simulink model "s9_template"  (R2023b)
settings: Solver=ode4  StartTime=0.0  StopTime=inf  FixedStep=P_sim_dt  RelTol=1e-3
InitFcn:
  | %madctrl_data;
  | s6_data;
values from neighbouring files (symbols this model uses):
  a1total = 2.70    (= 2.7)    [s6_data.m]
  a2total = 1.8    [s6_data.m]
  CarInputsCmdForward = uint8(1)    [p_mad_car.m]
  CarInputsCmdHalt = uint8(0)    [p_mad_car.m]
  CarInputsCmdReverse = uint8(2)    [p_mad_car.m]
  CarInputsCmdSlow = uint8(3)    [p_mad_car.m]
  P_k_p = 1    [s6_data.m]
  P_kr = 0.3440    (= 0.344)    [s6_data.m]
  P_ManeuverTypePark = 1    [s6_data.m]
  P_ManeuverTypePathFollow = 0    [s6_data.m]
  P_p_Bf = 0.7    [p_mad_car.m]
  P_p_Br = 0.7    [p_mad_car.m]
  P_p_Cf = 2    [p_mad_car.m]
  P_p_Cr = 2    [p_mad_car.m]
  P_p_delta_max = 21.58/180*pi    (= 0.37664205258)    [p_mad_car.m]
  P_p_Df = 2    [p_mad_car.m]
  P_p_Dr = 2.5    [p_mad_car.m]
  P_p_Ef = -0.1    [p_mad_car.m]
  P_p_Er = -0.05    [p_mad_car.m]
  P_p_J = 192e-6    (= 0.000192)    [p_mad_car.m]
  P_p_k = 2.51    [p_mad_car.m]
  P_p_l = abs(P_p_frontaxle_1 + P_p_rearaxle_1)    [p_mad_car.m]
  P_p_lf = P_p_frontaxle_1    (= 0.05)    [p_mad_car.m]
  P_p_lr = P_p_rearaxle_1    (= 0.049)    [p_mad_car.m]
  P_p_m = 132e-3    (= 0.132)    [p_mad_car.m]
  P_p_own = [P_p_s10; P_p_s20; 0; 0; 0; 0; 0 ]    [p_mad_car.m]
  P_p_T = 316e-3    (= 0.316)    [p_mad_car.m]
  P_p_Tt = P_p_uTt + P_p_output_Tt    (= 0.1)    [p_mad_car.m]
  P_p_Tw = 300e-3    (= 0.3)    [s6_data.m]
  P_prevent_buffer = 0.1    [s6_data.m]
  P_safety_buffer = 0.05    [s6_data.m]
  P_Ta = 20e-3    (= 0.02)    [s6_data.m]
  P_Ti = 0.2468    [s6_data.m]
  P_w_breakslen = uint32(length(path.points))    [s6_data.m]
  P_w_coefs = zeros(SPLINE.Elements(3).Dimensions)    [s6_data.m]
  P_w_points = zeros(SPLINE.Elements(2).Dimensions)    [s6_data.m]
  P_w_segments = uint32(zeros(SPLINE.Elements(4).Dimensions))    [s6_data.m]
  P_xManeuverEnd = 1    [s6_data.m]
  points = [p.x+x; s1; s2]    [mbc_clothoid_get_points.m]
undefined symbols (not defined in the file or in its folder): breakslen, coefs, DiscIntNeverNeededParam, periodic, segments
libraries: mad_lib_template x1, simulink x1
(part 1 of 2)
settings Model: Creator=hmekiedj  LastModifiedBy=Dominik
settings DataIOCC: ReturnWorkspaceOutputs=off
settings OptimizationCC: BlockReduction=off  DefaultParameterBehavior=Inlined  BufferReuse=off
settings DebuggingCC: UnconnectedInputMsg=warning  UnconnectedOutputMsg=warning  UnconnectedLineMsg=warning  ArithmeticOperatorsInVariantConditions=warning
settings ModelReferenceCC: EnableRefExpFcnMdlSchedulingChecks=on
settings SFSimCC: SimUseLocalCustomCode=off  CustomCodeUndefinedFunction=UseInterfaceOnly
settings RTWCC: RTWUseLocalCustomCode=off  DLArmComputeVersion=19.05
settings CodeAppCC: StateflowObjectComments=on

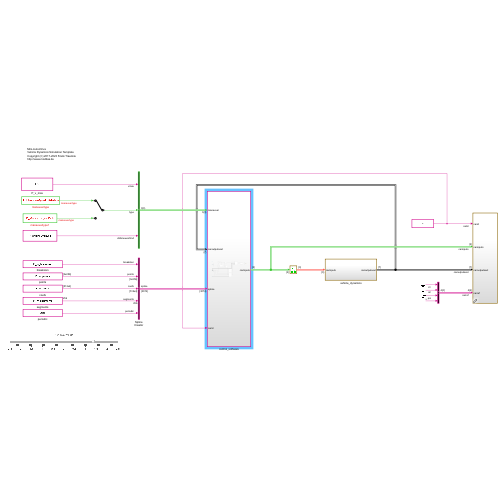
[thumbnail: Simulink's stored preview of the top-level diagram]
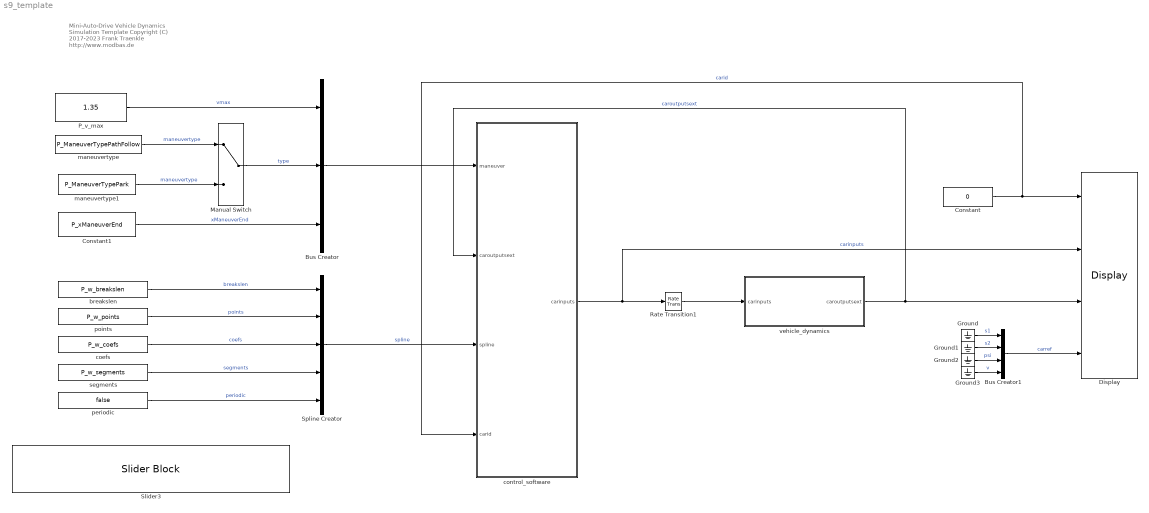
== system s9_template ==
  note: Mini-Auto-Drive
      | Vehicle Dynamics Simulation Template
      | Copyright (C) 2017-2023 Frank Traenkle
      | http://www.modbas.de
  Bus Creator : BusCreator  Inputs=3
  Bus Creator1 : BusCreator  Inputs=4
  Constant : Constant  Value=0
  Constant1 : Constant  Value=P_xManeuverEnd
  Display : mad_lib_template/Display  SystemSampleTime=-1  VariantActivationTime=update diagram  AllowFlexibleInterface=on  Latency=0  AutoFrameSizeCalculation=off
  Ground{,1..3} (4 alike) : Ground
  Manual Switch : ManualSwitch
  P_v_max : Constant  Value=1.35
  Rate Transition1 : RateTransition
  Slider3 : SliderBlock  ScaleMin=-2.50  ScaleMax=2.50  TickInterval=0.5
  Spline Creator : BusCreator  Inputs=breakslen,points,coefs,segments,periodic  OutDataTypeStr=Bus: SPLINE
  breakslen : Constant  Value=P_w_breakslen
  coefs : Constant  Value=P_w_coefs
  control_software : Subsystem  TreatAsAtomicUnit=on  SystemSampleTime=P_Ta
  maneuvertype : Constant  Value=P_ManeuverTypePathFollow  SampleTime=-1
  maneuvertype1 : Constant  Value=P_ManeuverTypePark  SampleTime=-1
  periodic : Constant  Value=false
  points : Constant  Value=P_w_points
  segments : Constant  Value=P_w_segments
  vehicle_dynamics : Subsystem
  wires:
  Bus Creator1/1 -> Display/4  "carref"
  Ground/1 -> Bus Creator1/1  "s1"
  Ground1/1 -> Bus Creator1/2  "s2"
  Ground2/1 -> Bus Creator1/3  "psi"
  Ground3/1 -> Bus Creator1/4  "v"
  vehicle_dynamics/1(caroutputsext) -> control_software/2(caroutputsext), Display/3  "caroutputsext"
  Rate Transition1/1 -> vehicle_dynamics/1(carinputs)
  control_software/1(carinputs) -> Display/2, Rate Transition1/1  "carinputs"
  Bus Creator/1 -> control_software/1(maneuver)
  P_v_max/1 -> Bus Creator/1  "vmax"
  Manual Switch/1 -> Bus Creator/2  "type"
  maneuvertype/1 -> Manual Switch/1  "maneuvertype"
  maneuvertype1/1 -> Manual Switch/2  "maneuvertype"
  Constant1/1 -> Bus Creator/3  "xManeuverEnd"
  periodic/1 -> Spline Creator/5  "periodic"
  coefs/1 -> Spline Creator/3  "coefs"
  points/1 -> Spline Creator/2  "points"
  breakslen/1 -> Spline Creator/1  "breakslen"
  segments/1 -> Spline Creator/4  "segments"
  Spline Creator/1 -> control_software/3(spline)  "spline"
  Constant/1 -> Display/1, control_software/4(carid)  "carid"

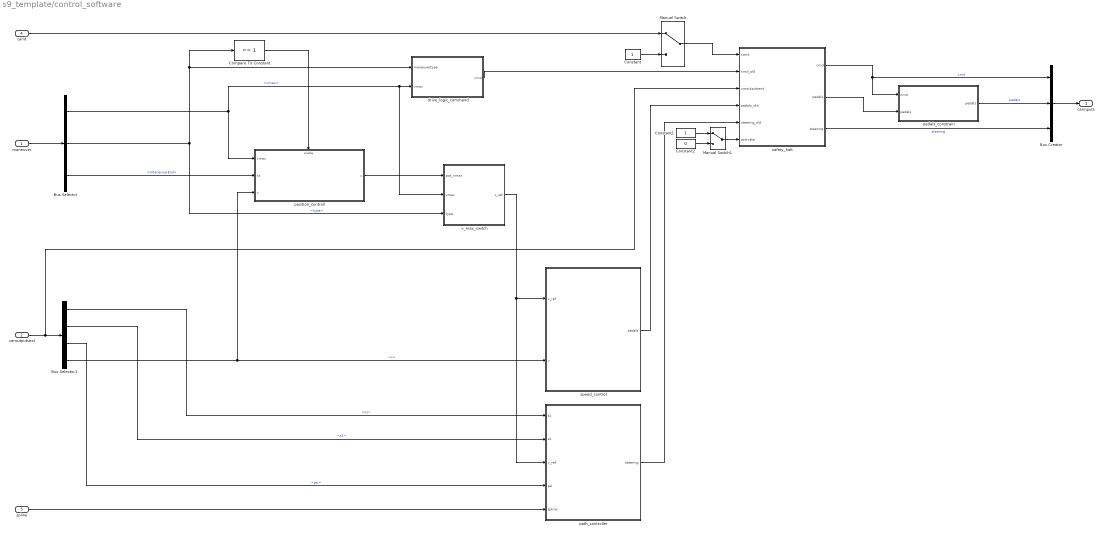
== system s9_template/control_software ==
  maneuver : Inport
  caroutputsext : Inport  Port=2
  spline : Inport  Port=3
  carid : Inport  Port=4
  Bus Creator : BusCreator  Inputs=3
  Bus Selector : BusSelector  OutputSignals=vmax,type,xManeuverEnd
  Bus Selector1 : BusSelector  OutputSignals=s1,s2,psi,v
  Compare To Constant : simulink/Logic and Bit Operations/Compare To Constant  relop===  const=1  OutDataTypeStr=boolean
  Constant : Constant
  Constant1 : Constant
  Constant2 : Constant  Value=0
  Manual Switch : ManualSwitch
  Manual Switch1 : ManualSwitch
  drive_logic_command : MATLAB Function  TreatAsAtomicUnit=on
  path_controller : Subsystem
  pedals_constrain : MATLAB Function  TreatAsAtomicUnit=on
  position_controll : Subsystem  TreatAsAtomicUnit=on
  safety_halt : MATLAB Function  TreatAsAtomicUnit=on
  speed_control : Subsystem
  v_max_switch : MATLAB Function  TreatAsAtomicUnit=on
  carinputs : Outport
  wires:
  caroutputsext/1 -> safety_halt/3(caroutputsext), Bus Selector1/1
  position_controll/1(u) -> v_max_switch/1(pos_vmax)
  maneuver/1 -> Bus Selector/1
  Bus Selector/1 -> position_controll/1(vmax), v_max_switch/2(vmax), drive_logic_command/2(vmax)  "<vmax>"
  Bus Selector/2 -> v_max_switch/3(type), Compare To Constant/1, drive_logic_command/1(maneuvertype)  "<type>"
  Compare To Constant/1 -> position_controll/Enable
  Bus Creator/1 -> carinputs/1
  Bus Selector/3 -> position_controll/2(xs)  "<xManeuverEnd>"
  drive_logic_command/1(cmd) -> safety_halt/2(cmd_old)
  path_controller/1(steering) -> safety_halt/5(steering_old)
  spline/1 -> path_controller/5(spline)
  safety_halt/1(cmd) -> pedals_constrain/1(cmd), Bus Creator/1  "cmd"
  carid/1 -> Manual Switch/1
  Bus Selector1/1 -> path_controller/1(s1)  "<s1>"
  Bus Selector1/2 -> path_controller/2(s2)  "<s2>"
  Bus Selector1/3 -> path_controller/4(psi)  "<psi>"
  Bus Selector1/4 -> position_controll/3(v), speed_control/2(v)  "<v>"
  Constant/1 -> Manual Switch/2
  Manual Switch/1 -> safety_halt/1(carid)
  v_max_switch/1(v_ref) -> path_controller/3(v_ref), speed_control/1(v_ref)
  speed_control/1(pedals) -> safety_halt/4(pedals_old)
  pedals_constrain/1(pedals) -> Bus Creator/2  "pedals"
  safety_halt/3(steering) -> Bus Creator/3  "steering"
  safety_halt/2(pedals) -> pedals_constrain/2("pedals ")
  Constant1/1 -> Manual Switch1/1
  Constant2/1 -> Manual Switch1/2
  Manual Switch1/1 -> safety_halt/6(activate)

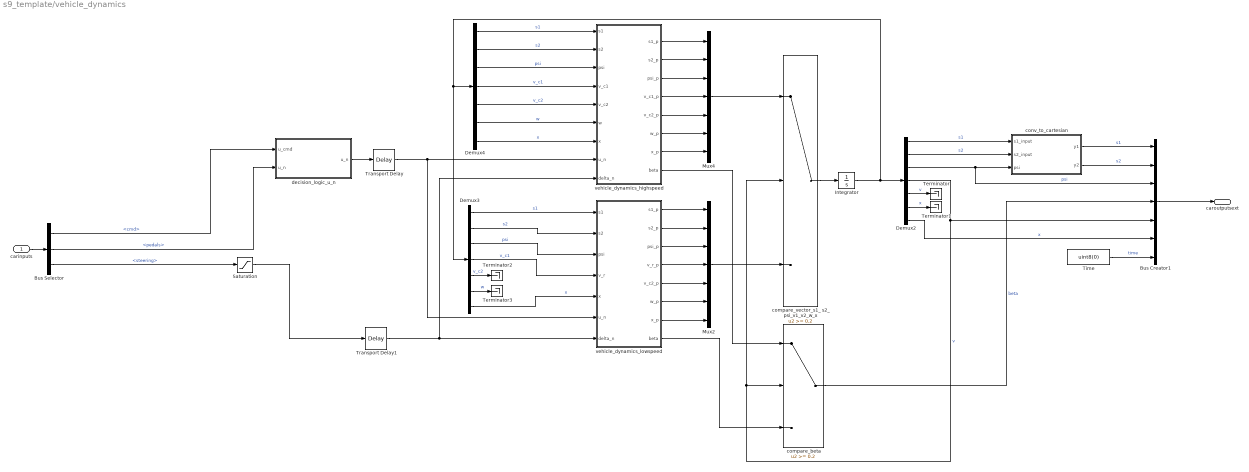
== system s9_template/vehicle_dynamics ==
  carinputs : Inport
  Bus Creator1 : BusCreator  Inputs=7  OutDataTypeStr=Bus: CAROUTPUTSEXT
  Bus Selector : BusSelector  OutputSignals=cmd,pedals,steering
  Demux2 : Demux  Outputs=7
  Demux3 : Demux  Outputs=7
  Demux4 : Demux  Outputs=7
  Integrator : Integrator  InitialCondition=P_p_own
  Mux2 : Mux  Inputs=7
  Mux4 : Mux  Inputs=7
  Saturation : Saturate  UpperLimit=1  LowerLimit=-1
  Terminator{,1..3} (4 alike) : Terminator
  Time : Constant  Value=uint8(0)
  Transport Delay : TransportDelay  DelayTime=P_p_Tt
  Transport Delay1 : TransportDelay  DelayTime=P_p_Tt
  compare_beta : Switch  Threshold=0.2  SaturateOnIntegerOverflow=off  InputSameDT=off
  compare_vector_s1_ s2_psi_v1_v2_w_x : Switch  Threshold=0.2  SaturateOnIntegerOverflow=off  InputSameDT=off
  conv_to_cartesian : MATLAB Function  TreatAsAtomicUnit=on
  decision_logic_u_n : MATLAB Function  TreatAsAtomicUnit=on
  vehicle_dynamics_highspeed : Subsystem
  vehicle_dynamics_lowspeed : Subsystem
  caroutputsext : Outport  VectorParamsAs1DForOutWhenUnconnected=off
  wires:
  carinputs/1 -> Bus Selector/1
  Bus Selector/2 -> decision_logic_u_n/2("u_n ")  "<pedals>"
  Bus Selector/3 -> Saturation/1  "<steering>"
  Demux2/3 -> conv_to_cartesian/3(psi), Bus Creator1/3  "psi"
  Bus Creator1/1 -> caroutputsext/1
  Demux2/7 -> Bus Creator1/6  "x"
  Demux2/2 -> conv_to_cartesian/2(s2_input)  "s2"
  Demux2/1 -> conv_to_cartesian/1(s1_input)  "s1"
  Bus Selector/1 -> decision_logic_u_n/1(u_cmd)  "<cmd>"
  Saturation/1 -> Transport Delay1/1
  vehicle_dynamics_highspeed/1(s1_p) -> Mux4/1
  vehicle_dynamics_highspeed/2(s2_p) -> Mux4/2
  vehicle_dynamics_highspeed/3(psi_p) -> Mux4/3
  vehicle_dynamics_highspeed/4(v_c1_p) -> Mux4/4
  vehicle_dynamics_highspeed/5(v_c2_p) -> Mux4/5
  vehicle_dynamics_highspeed/6(w_p) -> Mux4/6
  vehicle_dynamics_highspeed/7(x_p) -> Mux4/7
  vehicle_dynamics_lowspeed/1(s1_p) -> Mux2/1
  vehicle_dynamics_lowspeed/2(s2_p) -> Mux2/2
  vehicle_dynamics_lowspeed/3(psi_p) -> Mux2/3
  vehicle_dynamics_lowspeed/4(v_r_p) -> Mux2/4
  vehicle_dynamics_lowspeed/5(v_c2_p) -> Mux2/5
  vehicle_dynamics_lowspeed/6(w_p) -> Mux2/6
  vehicle_dynamics_lowspeed/7(x_p) -> Mux2/7
  Mux4/1 -> compare_vector_s1_ s2_psi_v1_v2_w_x/1
  compare_vector_s1_ s2_psi_v1_v2_w_x/1 -> Integrator/1
  Integrator/1 -> Demux2/1, Demux4/1, Demux3/1
  Demux2/4 -> compare_vector_s1_ s2_psi_v1_v2_w_x/2, compare_beta/2, Bus Creator1/5  "v"
  Demux3/1 -> vehicle_dynamics_lowspeed/1(s1)  "s1"
  Demux3/2 -> vehicle_dynamics_lowspeed/2(s2)  "s2"
  Demux3/3 -> vehicle_dynamics_lowspeed/3(psi)  "psi"
  Demux3/4 -> vehicle_dynamics_lowspeed/4(v_r)  "v_c1"
  Demux3/7 -> vehicle_dynamics_lowspeed/5(x)  "x"
  Demux4/1 -> vehicle_dynamics_highspeed/1(s1)  "s1"
  Demux4/2 -> vehicle_dynamics_highspeed/2(s2)  "s2"
  Demux4/3 -> vehicle_dynamics_highspeed/3(psi)  "psi"
  Demux4/4 -> vehicle_dynamics_highspeed/4(v_c1)  "v_c1"
  Demux4/5 -> vehicle_dynamics_highspeed/5(v_c2)  "v_c2"
  Demux4/6 -> vehicle_dynamics_highspeed/6(w)  "w"
  Demux4/7 -> vehicle_dynamics_highspeed/7(x)  "x"
  Transport Delay/1 -> vehicle_dynamics_lowspeed/6(u_n), vehicle_dynamics_highspeed/8(u_n)
  Transport Delay1/1 -> vehicle_dynamics_lowspeed/7(delta_n), vehicle_dynamics_highspeed/9(delta_n)
  vehicle_dynamics_lowspeed/8(beta) -> compare_beta/3
  vehicle_dynamics_highspeed/8(beta) -> compare_beta/1
  compare_beta/1 -> Bus Creator1/4  "beta"
  conv_to_cartesian/1(y1) -> Bus Creator1/1  "s1"
  conv_to_cartesian/2(y2) -> Bus Creator1/2  "s2"
  Demux2/5 -> Terminator/1  "v"
  Demux2/6 -> Terminator1/1  "x"
  decision_logic_u_n/1(u_n) -> Transport Delay/1
  Demux3/5 -> Terminator2/1  "v_c2"
  Demux3/6 -> Terminator3/1  "w"
  Mux2/1 -> compare_vector_s1_ s2_psi_v1_v2_w_x/3
  Time/1 -> Bus Creator1/7  "time"

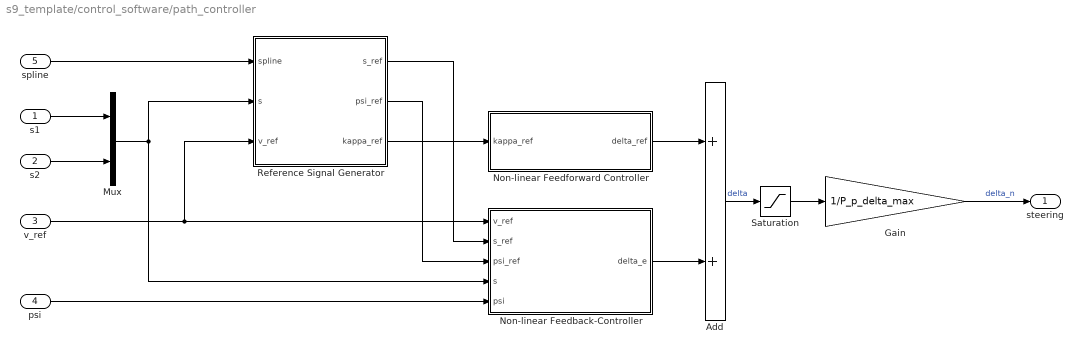
== system s9_template/control_software/path_controller ==
  s1 : Inport
  s2 : Inport  Port=2
  v_ref : Inport  Port=3
  psi : Inport  Port=4
  spline : Inport  Port=5
  Add : Sum
  Gain : Gain  Gain=1/P_p_delta_max
  Mux : Mux  Inputs=2
  Non-linear Feedback-Controller : MATLAB Function  TreatAsAtomicUnit=on
  Non-linear Feedforward Controller : MATLAB Function  TreatAsAtomicUnit=on
  Reference Signal Generator : MATLAB Function  TreatAsAtomicUnit=on
  Saturation : Saturate  UpperLimit=1  LowerLimit=-1
  steering : Outport
  wires:
  spline/1 -> Reference Signal Generator/1(spline)
  s1/1 -> Mux/1
  s2/1 -> Mux/2
  v_ref/1 -> Reference Signal Generator/3(v_ref), Non-linear Feedback-Controller/1(v_ref)
  Reference Signal Generator/3(kappa_ref) -> Non-linear Feedforward Controller/1(kappa_ref)
  Reference Signal Generator/2(psi_ref) -> Non-linear Feedback-Controller/3(psi_ref)
  Reference Signal Generator/1(s_ref) -> Non-linear Feedback-Controller/2(s_ref)
  Non-linear Feedforward Controller/1(delta_ref) -> Add/1
  Non-linear Feedback-Controller/1(delta_e) -> Add/2
  Add/1 -> Saturation/1  "delta"
  Gain/1 -> steering/1  "delta_n"
  Mux/1 -> Reference Signal Generator/2(s), Non-linear Feedback-Controller/4(s)
  psi/1 -> Non-linear Feedback-Controller/5(psi)
  Saturation/1 -> Gain/1

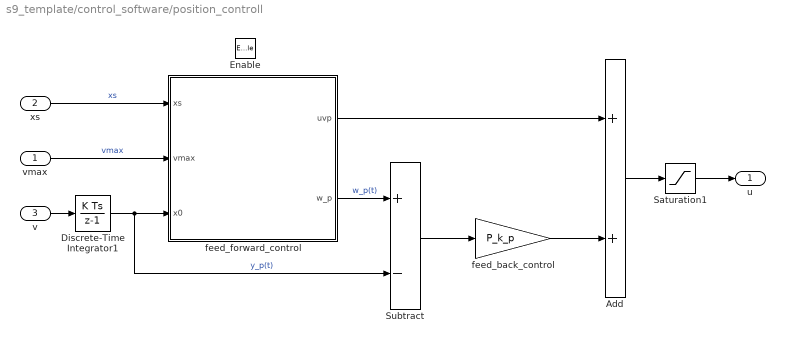
== system s9_template/control_software/position_controll ==
  vmax : Inport
  xs : Inport  Port=2
  v : Inport  Port=3
  Enable : EnablePort
  Add : Sum
  Discrete-Time Integrator1 : DiscreteIntegrator  SampleTime=-1  ICPrevOutput=DiscIntNeverNeededParam  ICPrevScaledInput=DiscIntNeverNeededParam
  Saturation1 : Saturate  UpperLimit=2.51  LowerLimit=-2.51
  Subtract : Sum  Inputs=+-
  feed_back_control : Gain  Gain=P_k_p
  feed_forward_control : Subsystem
  u : Outport
  wires:
  xs/1 -> feed_forward_control/1(xs)  "xs"
  feed_forward_control/2(w_p) -> Subtract/1  "w_p(t)"
  Subtract/1 -> feed_back_control/1
  feed_forward_control/1(uvp) -> Add/1
  vmax/1 -> feed_forward_control/2(vmax)  "vmax"
  feed_back_control/1 -> Add/2
  Add/1 -> Saturation1/1
  v/1 -> Discrete-Time Integrator1/1
  Saturation1/1 -> u/1
  Discrete-Time Integrator1/1 -> feed_forward_control/3(x0), Subtract/2  "y_p(t)"

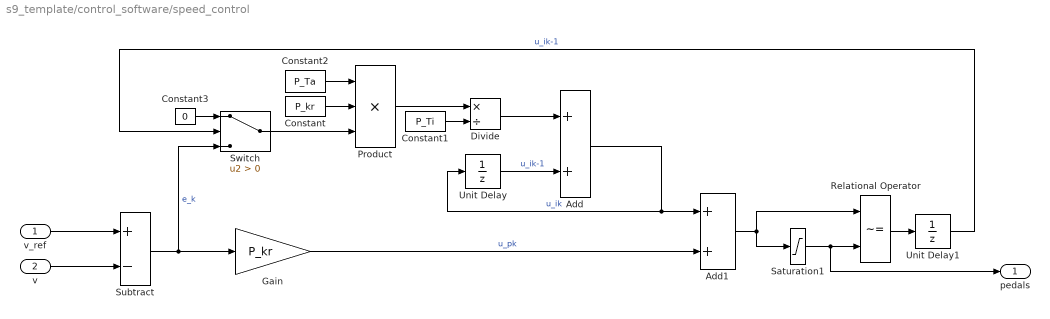
== system s9_template/control_software/speed_control ==
  v_ref : Inport
  v : Inport  Port=2
  Add : Sum
  Add1 : Sum
  Constant : Constant  Value=P_kr
  Constant1 : Constant  Value=P_Ti  VectorParams1D=off
  Constant2 : Constant  Value=P_Ta  VectorParams1D=off
  Constant3 : Constant  Value=0
  Divide : Product  Inputs=*/
  Gain : Gain  Gain=P_kr
  Product : Product  Inputs=3
  Relational Operator : RelationalOperator  Operator=~=  OutDataTypeStr=boolean  RndMeth=Simplest  InputSameDT=off
  Saturation1 : Saturate  UpperLimit=1  LowerLimit=-1
  Subtract : Sum  Inputs=+-
  Switch : Switch  Criteria=u2 > Threshold  SaturateOnIntegerOverflow=off  InputSameDT=off
  Unit Delay : UnitDelay  SampleTime=P_Ta  HasFrameUpgradeWarning=on
  Unit Delay1 : UnitDelay  SampleTime=P_Ta  HasFrameUpgradeWarning=on
  pedals : Outport
  wires:
  Constant3/1 -> Switch/1
  Relational Operator/1 -> Unit Delay1/1
  Divide/1 -> Add/1
  Subtract/1 -> Gain/1, Switch/3  "e_k"
  Constant2/1 -> Product/1
  Saturation1/1 -> Relational Operator/2, pedals/1
  Switch/1 -> Product/3
  Constant/1 -> Product/2
  Constant1/1 -> Divide/2
  Product/1 -> Divide/1
  Unit Delay1/1 -> Switch/2  "u_ik-1"
  Gain/1 -> Add1/2  "u_pk"
  Unit Delay/1 -> Add/2  "u_ik-1"
  Add/1 -> Add1/1, Unit Delay/1  "u_ik"
  Add1/1 -> Relational Operator/1, Saturation1/1
  v_ref/1 -> Subtract/1
  v/1 -> Subtract/2

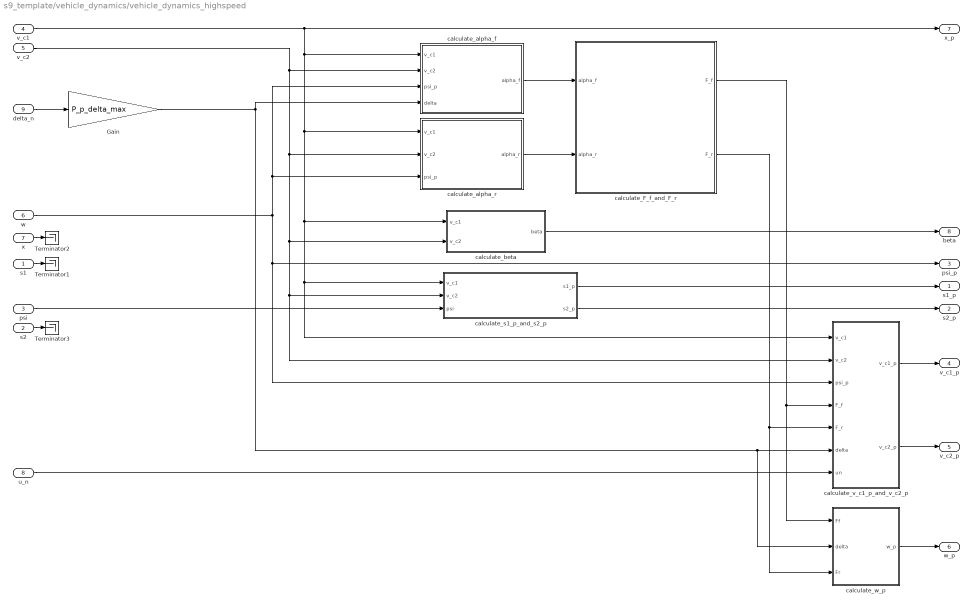
== system s9_template/vehicle_dynamics/vehicle_dynamics_highspeed ==
  s1 : Inport
  s2 : Inport  Port=2
  psi : Inport  Port=3
  v_c1 : Inport  Port=4
  v_c2 : Inport  Port=5
  w : Inport  Port=6
  x : Inport  Port=7
  u_n : Inport  Port=8
  delta_n : Inport  Port=9
  Gain : Gain  Gain=P_p_delta_max
  Terminator1 : Terminator
  Terminator2 : Terminator
  Terminator3 : Terminator
  calculate_F_f_and_F_r : MATLAB Function  TreatAsAtomicUnit=on
  calculate_alpha_f : MATLAB Function  TreatAsAtomicUnit=on
  calculate_alpha_r : MATLAB Function  TreatAsAtomicUnit=on
  calculate_beta : MATLAB Function  TreatAsAtomicUnit=on
  calculate_s1_p_and_s2_p : MATLAB Function  TreatAsAtomicUnit=on
  calculate_v_c1_p_and_v_c2_p : MATLAB Function  TreatAsAtomicUnit=on
  calculate_w_p : MATLAB Function  TreatAsAtomicUnit=on
  s1_p : Outport  VectorParamsAs1DForOutWhenUnconnected=off
  s2_p : Outport  Port=2  VectorParamsAs1DForOutWhenUnconnected=off
  psi_p : Outport  Port=3  VectorParamsAs1DForOutWhenUnconnected=off
  v_c1_p : Outport  Port=4  VectorParamsAs1DForOutWhenUnconnected=off
  v_c2_p : Outport  Port=5  VectorParamsAs1DForOutWhenUnconnected=off
  w_p : Outport  Port=6  VectorParamsAs1DForOutWhenUnconnected=off
  x_p : Outport  Port=7  VectorParamsAs1DForOutWhenUnconnected=off
  beta : Outport  Port=8  VectorParamsAs1DForOutWhenUnconnected=off
  wires:
  delta_n/1 -> Gain/1
  calculate_alpha_f/1(alpha_f) -> calculate_F_f_and_F_r/1(alpha_f)
  calculate_alpha_r/1(alpha_r) -> calculate_F_f_and_F_r/2(alpha_r)
  calculate_beta/1(beta) -> beta/1
  calculate_s1_p_and_s2_p/1(s1_p) -> s1_p/1
  calculate_s1_p_and_s2_p/2(s2_p) -> s2_p/1
  Gain/1 -> calculate_v_c1_p_and_v_c2_p/6(delta), calculate_w_p/2(delta), calculate_alpha_f/4(delta)
  w/1 -> psi_p/1, calculate_v_c1_p_and_v_c2_p/3(psi_p), calculate_alpha_r/3(psi_p), calculate_alpha_f/3(psi_p)
  u_n/1 -> calculate_v_c1_p_and_v_c2_p/7(un)
  calculate_F_f_and_F_r/2(F_r) -> calculate_w_p/3(Fr), calculate_v_c1_p_and_v_c2_p/5(F_r)
  calculate_F_f_and_F_r/1(F_f) -> calculate_w_p/1(Ff), calculate_v_c1_p_and_v_c2_p/4(F_f)
  calculate_v_c1_p_and_v_c2_p/1(v_c1_p) -> v_c1_p/1
  calculate_v_c1_p_and_v_c2_p/2(v_c2_p) -> v_c2_p/1
  v_c1/1 -> calculate_v_c1_p_and_v_c2_p/1(v_c1), calculate_s1_p_and_s2_p/1(v_c1), calculate_beta/1(v_c1), calculate_alpha_r/1(v_c1), calculate_alpha_f/1(v_c1), x_p/1
  v_c2/1 -> calculate_v_c1_p_and_v_c2_p/2(v_c2), calculate_s1_p_and_s2_p/2(v_c2), calculate_beta/2(v_c2), calculate_alpha_r/2(v_c2), calculate_alpha_f/2(v_c2)
  calculate_w_p/1(w_p) -> w_p/1
  psi/1 -> calculate_s1_p_and_s2_p/3(psi)
  x/1 -> Terminator2/1
  s1/1 -> Terminator1/1
  s2/1 -> Terminator3/1

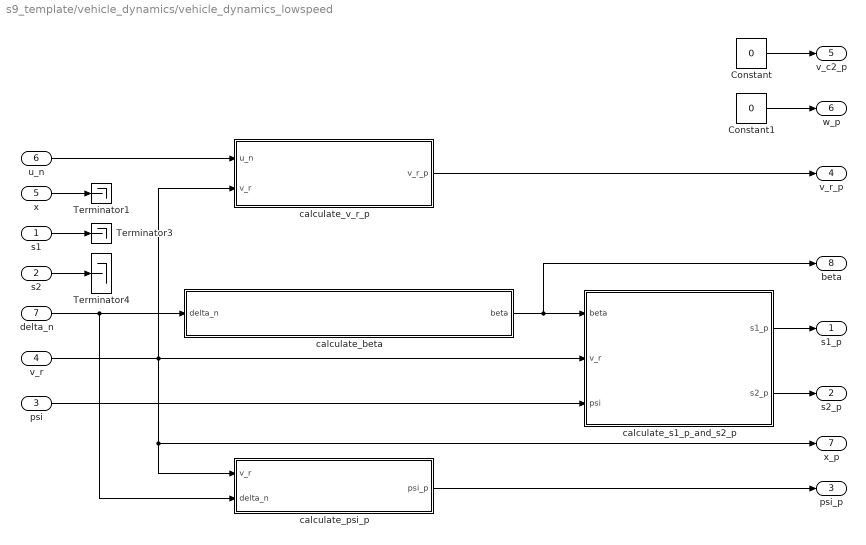
== system s9_template/vehicle_dynamics/vehicle_dynamics_lowspeed ==
  s1 : Inport
  s2 : Inport  Port=2
  psi : Inport  Port=3
  v_r : Inport  Port=4
  x : Inport  Port=5
  u_n : Inport  Port=6
  delta_n : Inport  Port=7
  Constant : Constant  Value=0
  Constant1 : Constant  Value=0
  Terminator1 : Terminator
  Terminator3 : Terminator
  Terminator4 : Terminator
  calculate_beta : Subsystem
  calculate_psi_p : Subsystem
  calculate_s1_p_and_s2_p : Subsystem
  calculate_v_r_p : Subsystem
  s1_p : Outport  VectorParamsAs1DForOutWhenUnconnected=off
  s2_p : Outport  Port=2  VectorParamsAs1DForOutWhenUnconnected=off
  psi_p : Outport  Port=3  VectorParamsAs1DForOutWhenUnconnected=off
  v_r_p : Outport  Port=4  VectorParamsAs1DForOutWhenUnconnected=off
  v_c2_p : Outport  Port=5  VectorParamsAs1DForOutWhenUnconnected=off
  w_p : Outport  Port=6  VectorParamsAs1DForOutWhenUnconnected=off
  x_p : Outport  Port=7  VectorParamsAs1DForOutWhenUnconnected=off
  beta : Outport  Port=8  VectorParamsAs1DForOutWhenUnconnected=off
  wires:
  u_n/1 -> calculate_v_r_p/1(u_n)
  calculate_v_r_p/1(v_r_p) -> v_r_p/1
  v_r/1 -> calculate_psi_p/1(v_r), x_p/1, calculate_s1_p_and_s2_p/2(v_r), calculate_v_r_p/2(v_r)
  delta_n/1 -> calculate_psi_p/2(delta_n), calculate_beta/1(delta_n)
  calculate_s1_p_and_s2_p/1(s1_p) -> s1_p/1
  psi/1 -> calculate_s1_p_and_s2_p/3(psi)
  calculate_beta/1(beta) -> calculate_s1_p_and_s2_p/1(beta), beta/1
  calculate_s1_p_and_s2_p/2(s2_p) -> s2_p/1
  calculate_psi_p/1(psi_p) -> psi_p/1
  x/1 -> Terminator1/1
  s1/1 -> Terminator3/1
  s2/1 -> Terminator4/1
  Constant/1 -> v_c2_p/1
  Constant1/1 -> w_p/1

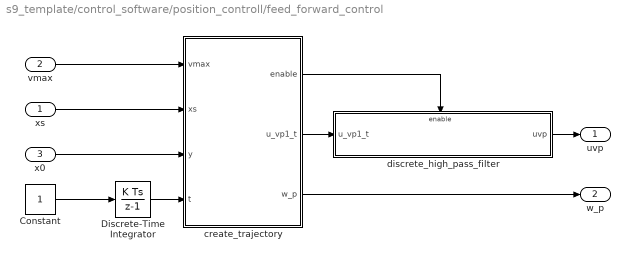
== system s9_template/control_software/position_controll/feed_forward_control ==
  xs : Inport
  vmax : Inport  Port=2
  x0 : Inport  Port=3
  Constant : Constant
  Discrete-Time Integrator : DiscreteIntegrator  SampleTime=-1  ICPrevOutput=DiscIntNeverNeededParam  ICPrevScaledInput=DiscIntNeverNeededParam
  "create_trajectory " : MATLAB Function  TreatAsAtomicUnit=on
  discrete_high_pass_filter : Subsystem  TreatAsAtomicUnit=on
  uvp : Outport
  w_p : Outport  Port=2
  wires:
  x0/1 -> "create_trajectory "/3(y)
  vmax/1 -> "create_trajectory "/1(vmax)
  xs/1 -> "create_trajectory "/2(xs)
  "create_trajectory "/3(w_p) -> w_p/1
  Constant/1 -> Discrete-Time Integrator/1
  Discrete-Time Integrator/1 -> "create_trajectory "/4(t)
  "create_trajectory "/2(u_vp1_t) -> discrete_high_pass_filter/1(u_vp1_t)
  discrete_high_pass_filter/1(uvp) -> uvp/1
  "create_trajectory "/1(enable) -> discrete_high_pass_filter/Enable

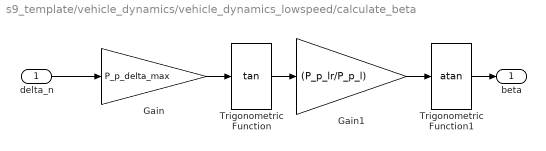
== system s9_template/vehicle_dynamics/vehicle_dynamics_lowspeed/calculate_beta ==
  delta_n : Inport
  Gain : Gain  Gain=P_p_delta_max
  Gain1 : Gain  Gain=(P_p_lr/P_p_l)
  Trigonometric Function : Trigonometry  Operator=tan
  Trigonometric Function1 : Trigonometry  Operator=atan
  beta : Outport  VectorParamsAs1DForOutWhenUnconnected=off
  wires:
  delta_n/1 -> Gain/1
  Gain/1 -> Trigonometric Function/1
  Trigonometric Function/1 -> Gain1/1
  Gain1/1 -> Trigonometric Function1/1
  Trigonometric Function1/1 -> beta/1

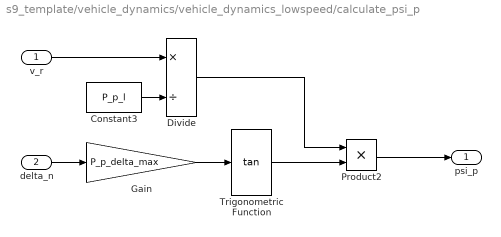
== system s9_template/vehicle_dynamics/vehicle_dynamics_lowspeed/calculate_psi_p ==
  v_r : Inport
  delta_n : Inport  Port=2
  Constant3 : Constant  Value=P_p_l
  Divide : Product  Inputs=*/
  Gain : Gain  Gain=P_p_delta_max
  Product2 : Product
  Trigonometric Function : Trigonometry  Operator=tan
  psi_p : Outport  VectorParamsAs1DForOutWhenUnconnected=off
  wires:
  delta_n/1 -> Gain/1
  Gain/1 -> Trigonometric Function/1
  Product2/1 -> psi_p/1
  v_r/1 -> Divide/1
  Constant3/1 -> Divide/2
  Trigonometric Function/1 -> Product2/2
  Divide/1 -> Product2/1

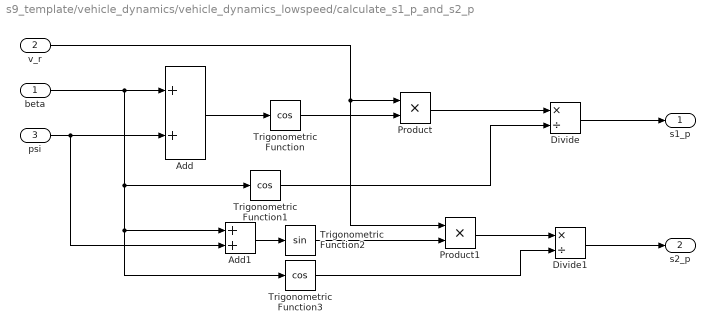
== system s9_template/vehicle_dynamics/vehicle_dynamics_lowspeed/calculate_s1_p_and_s2_p ==
  beta : Inport
  v_r : Inport  Port=2
  psi : Inport  Port=3
  Add : Sum
  Add1 : Sum
  Divide : Product  Inputs=*/
  Divide1 : Product  Inputs=*/
  Product : Product
  Product1 : Product
  Trigonometric Function : Trigonometry  Operator=cos
  Trigonometric Function1 : Trigonometry  Operator=cos
  Trigonometric Function2 : Trigonometry
  Trigonometric Function3 : Trigonometry  Operator=cos
  s1_p : Outport  VectorParamsAs1DForOutWhenUnconnected=off
  s2_p : Outport  Port=2  VectorParamsAs1DForOutWhenUnconnected=off
  wires:
  Add/1 -> Trigonometric Function/1
  Trigonometric Function/1 -> Product/2
  Product/1 -> Divide/1
  Trigonometric Function1/1 -> Divide/2
  Divide/1 -> s1_p/1
  psi/1 -> Add1/2, Add/2
  beta/1 -> Trigonometric Function1/1, Trigonometric Function3/1, Add1/1, Add/1
  Trigonometric Function2/1 -> Product1/2
  Divide1/1 -> s2_p/1
  v_r/1 -> Product1/1, Product/1
  Product1/1 -> Divide1/1
  Add1/1 -> Trigonometric Function2/1
  Trigonometric Function3/1 -> Divide1/2

== system s9_template/vehicle_dynamics/vehicle_dynamics_lowspeed/calculate_v_r_p ==
  u_n : Inport
  v_r : Inport  Port=2
  Add : Sum  Inputs=-+
  Gain : Gain  Gain=(1/P_p_T)
  Gain1 : Gain  Gain=(P_p_k/P_p_T)
  v_r_p : Outport  VectorParamsAs1DForOutWhenUnconnected=off
  wires:
  Gain/1 -> Add/1
  Add/1 -> v_r_p/1
  v_r/1 -> Gain/1
  u_n/1 -> Gain1/1
  Gain1/1 -> Add/2

== system s9_template/control_software/position_controll/feed_forward_control/discrete_high_pass_filter ==
  u_vp1_t : Inport
  Enable : EnablePort  StatesWhenEnabling=reset
  discrete_high_pass_filter : DiscreteTransferFcn  Numerator=[2, -2]  Denominator=[(P_Ta+(2*P_Ti)), (P_Ta-(2*P_Ti))]
  uvp : Outport  OutputWhenDisabled=reset  InitialOutput=[0]
  wires:
  u_vp1_t/1 -> discrete_high_pass_filter/1
  discrete_high_pass_filter/1 -> uvp/1

== matlab function s9_template/vehicle_dynamics/vehicle_dynamics_highspeed/calculate_v_c1_p_and_v_c2_p ==
  data: v_c1 input; v_c1_p output; v_c2 input; psi_p input; v_c2_p output; F_f input; F_r input; delta input; un input; P_p_m parameter; P_p_T parameter; P_p_k parameter
function [v_c1_p, v_c2_p] = calculate_v_c1_p_and_v_c2_p(v_c1, v_c2, psi_p, F_f, F_r, delta, un, P_p_m, P_p_T, P_p_k)
    % Function: calculate_v_c1_p_and_v_c2_p
    % Description: Calculates the updated longitudinal and lateral velocity components 
    %              of a vehicle based on various dynamic parameters and forces.
    %
    % Inputs:
    %   v_c1 [m/s] - Initial longitudinal velocity component.
    %   v_c2 [m/s] - Initial lateral velocity component.
    %   psi_p [rad] - Yaw rate of the vehicle.
    %   F_f [N] - Tire force at the front of the vehicle.
    %   F_r [N] - Tire force at the rear of the vehicle.
    %   delta [rad] - Steering angle.
    %   un [1] - Motor control signal.
    %   P_p_m [kg] - Mass of the vehicle.
    %   P_p_T [s] - Time constant related to the vehicle dynamics.
    %   P_p_k [m/s] - Constant related to the motor control effectiveness.
    %
    % Outputs:
    %   v_c1_p [m/s] - Updated longitudinal velocity component.
    %   v_c2_p [m/s] - Updated lateral velocity component.
    %
    % The function calculates the new velocity components considering the external forces,
    % vehicle's yaw rate, steering angle, motor control signal, and various vehicle parameters.
    % These calculations are essential for understanding the vehicle's dynamic behavior under
    % different control inputs and conditions.
    
    % Calculating the updated velocity components
    v_c1_p = double((1 / P_p_m) * (-F_f * sin(delta) + (P_p_m * v_c2 * psi_p)) - (1 / P_p_T * v_c1) + ((P_p_k / P_p_T) * un));
    v_c2_p = double((1 / P_p_m) * (F_f * cos(delta) + F_r - (P_p_m * v_c1 * psi_p)));
end

== matlab function s9_template/vehicle_dynamics/vehicle_dynamics_highspeed/calculate_w_p ==
  data: w_p output; Ff input; delta input; Fr input; P_p_J parameter; P_p_lf parameter; P_p_lr parameter
function w_p = calculate_w_p(Ff, delta, Fr, P_p_J, P_p_lf, P_p_lr)
    % Function: calculate_w_p
    % Description: Calculates the yaw rate change 'w_p' of a vehicle.
    %
    % Inputs:
    %   Ff [N] - Front tire force.
    %   delta [rad] - Steering angle.
    %   Fr [N] - Rear tire force.
    %   P_p_J [kg*m^2] - Moment of inertia of the vehicle about the yaw axis.
    %   P_p_lf [m] - Distance from the center of gravity (COG) to the front axle.
    %   P_p_lr [m] - Distance from the COG to the rear axle.
    %
    % Output:
    %   w_p [rad] - Calculated change in yaw rate.
    %
    % The function computes the change in the vehicle's yaw rate based on the forces 
    % acting on the front and rear tires, the steering angle, the vehicle's moment of 
    % inertia, and the distances from the COG to the front and rear axles. This calculation 
    % is crucial for understanding the vehicle's dynamic response to steering inputs.
    
    % Calculation of the yaw rate change 'w_p'
    w_p = 1 / P_p_J * (Ff * P_p_lf * cos(delta) - Fr * P_p_lr);
end

== matlab function s9_template/control_software/drive_logic_command ==
  data: maneuvertype input; vmax input; cmd output; CarInputsCmdReverse parameter; CarInputsCmdForward parameter; CarInputsCmdSlow parameter
function cmd = drive_logic_command(maneuvertype, vmax, CarInputsCmdReverse, CarInputsCmdForward, CarInputsCmdSlow)
    % Function: fcn
    % Description: Determines the appropriate command for vehicle maneuver based on the 
    %              maneuver type and maximum velocity.
    %
    % Inputs:
    %   maneuvertype [1] - Numeric value indicating the type of maneuver.
    %   vmax [m/s]- Maximum velocity 
    %   CarInputsCmdReverse [1] - Command for reversing the vehicle.
    %   CarInputsCmdForward [1]- Command for moving the vehicle forward.
    %   CarInputsCmdSlow [1] - Command for slowing down the vehicle.
    %
    % Output:
    %   cmd [1] - The calculated command for the vehicle maneuver.
    %
    % The function sets the command for a vehicle maneuver based on the maneuver type and 
    % maximum velocity. If the maneuver type is 1, it sets the command to slow down. Otherwise, 
    % it chooses between moving forward or reversing based on the maximum velocity.

    % Setting the initial command to forward
    cmd = CarInputsCmdForward;
    
    % Logic to determine the command based on maneuver type and maximum velocity
    if maneuvertype == 1
        cmd = CarInputsCmdSlow;
    else
        if vmax >= 0
            cmd = CarInputsCmdForward;
        elseif vmax < 0
            cmd = CarInputsCmdReverse;
        end 
    end
end

== matlab function s9_template/control_software/path_controller/Reference Signal Generator ==
  data: spline input; s_ref output; s input size=2; v_ref input size=1; psi_ref output; kappa_ref output; P_p_Tt parameter
function [s_ref, psi_ref, kappa_ref] = E_ref(spline, s, v_ref, P_p_Tt)
    % Function: E_ref
    % Description: Calculates reference values for position, orientation, and curvature
    %              based on a given spline, position, and velocity.
    %
    % Inputs:
    %   spline [1] - Spline structure containing points, coefficients, lengths, and periodicity.
    %   s [1] - Current position along the spline.
    %   v_ref [m/s] - Reference velocity.
    %   P_p_Tt [s] - Dead time affecting the response.
    %
    % Outputs:
    %   s_ref [1] - Reference position in terms of x and y coordinates.
    %   psi_ref [rad] - Reference orientation (yaw angle).
    %   kappa_ref [1/m] - Reference curvature.
    %
    % The function uses the spline data along with the current position and reference velocity
    % to determine the reference position (s_ref), orientation (psi_ref), and curvature (kappa_ref).
    % These are crucial for path following and trajectory planning in vehicle dynamics.
    %
    % Extracting spline components
    points = spline.points;
    coefs = spline.coefs;
    breakslen = spline.breakslen;
    periodic = spline.periodic;
    
    % Calculating reference values using spline data
    [w, widx] = mbc_spline_get_reference(s, breakslen, points, coefs, periodic, v_ref, P_p_Tt);
    
    % Assigning the calculated reference values
    psi_ref = w(2);
    kappa_ref = w(5);
    s_ref = [w(3), w(4)];
end

== matlab function s9_template/control_software/path_controller/Non-linear Feedforward Controller ==
  data: kappa_ref input; delta_ref output; P_p_l parameter
function delta_ref = E_FF(kappa_ref, P_p_l)
    % Function: E_FF
    % Description: Calculates the reference steering angle 'delta_ref' for feedforward control.
    %
    % Inputs:
    %   kappa_ref [1/m] - Reference curvature of the path.
    %   P_p_l [m] - Wheelbase length of the vehicle.
    %
    % Output:
    %   delta_ref [rad] - Calculated reference steering angle for feedforward control.
    %
    % The function computes the reference steering angle (delta_ref) needed for a vehicle
    % to follow a path with a given curvature (kappa_ref). This calculation is crucial in
    % feedforward control systems where precise steering based on the path's curvature is required.
    %

    % Calculating the reference steering angle based on the curvature and wheelbase
    delta_ref = atan(P_p_l * kappa_ref);
end

== matlab function s9_template/control_software/path_controller/Non-linear Feedback-Controller ==
  data: v_ref input; delta_e output; s_ref input; psi_ref input; s input; psi input; P_p_Tw parameter; P_p_l parameter
function delta_e = E_FB(v_ref, s_ref, psi_ref, s, psi, P_p_Tw, P_p_l)
    % Function: E_FB
    % Description: Calculates the steering angle error 'delta_e' for feedback control in vehicle dynamics.
    %
    % Inputs:
    %   v_ref [m/s] - Reference velocity.
    %   s_ref [1] - Reference position coordinates (x_ref, y_ref).
    %   psi_ref [rad] - Reference orientation (yaw angle).
    %   s [1] - Current position coordinates (x, y).
    %   psi [rad] - Current orientation (yaw angle).
    %   P_p_Tw [s] - Time constant Tw.
    %   P_p_l [m] - Wheelbase length of the vehicle.
    %
    % Output:
    %   delta_e [rad] - Calculated error in steering angle.
    %
    % The function computes the error in the steering angle for feedback control. It first
    % normalizes the orientation error and calculates the lateral position error. The function
    % then adjusts the reference velocity if it's within a certain range for accuracy. Finally,
    % it uses these errors to calculate the steering angle error based on the vehicle's dynamics.

    % Calculate orientation error and normalize
    psi_e = psi - psi_ref;
    psi_e = mod(psi_e + pi, 2*pi) - pi;
    
    % Calculate lateral position error
    sc2_e = (s(2) - s_ref(2)) * cos(psi_ref) - (s(1) - s_ref(1)) * sin(psi_ref);
    
    % Adjust reference velocity for calculation
    v_e = 0.1;
    if v_ref > v_e || v_ref < -v_e
        v_ref = v_ref;
    elseif v_ref >= 0 && v_ref <= v_e
        v_ref = v_e;
    elseif v_ref >= -v_e && v_ref < 0
        v_ref = -v_e;
    end
    
    % Calculate steering angle error
    delta_e = -(P_p_l / (P_p_Tw^2 * v_ref^2)) * sc2_e - (2 * P_p_l / (P_p_Tw * v_ref)) * psi_e;
end

== matlab function s9_template/control_software/position_controll/feed_forward_control/create_trajectory  ==
  data: enable output; vmax input; u_vp1_t output; xs input; y input; w_p output; t input; P_p_k parameter; P_p_T parameter; P_p_Tt parameter; P_kr parameter; P_Ti parameter
function [enable, u_vp1_t, w_p] = create_trajectory (vmax, xs, y, t, P_p_k, P_p_T, P_p_Tt, P_kr, P_Ti)
    % Function: fcn
    % Description: Calculates control signals based on predefined reference polynomials
    %              and time-varying parameters.
    %
    % Inputs:
    %   vmax - Maximum velocity. [m/s]
    %   xs - Target state variable. [m]
    %   y - Initial state variable. [1]
    %   t - Current time. [s]
    %   P_p_k [m/s], P_p_T [s], P_p_Tt [s] - Parameters for the control dynamics.
    %   P_kr [s/m], P_Ti [s] - Parameters for the reference polynomial dynamics.
    %
    % Outputs:
    %   u_vp1_t - Control signal at time t.
    %   w_p - Reference polynomial value at time t.
    %
    % The function computes control signals based on a reference polynomial that is defined 
    % initially and a feedforward polynomial. It uses persistent variables to store the 
    % polynomial coefficients and evaluates them based on the current time 't'. This is useful 
    % for dynamic control systems where the control signal needs to adapt over time.
    
    % Initialize persistent variables if they are empty
    persistent c x0 te cff;
    if isempty(c)
        x0 = y;
        [c, te] = cd_refpoly_vmax(vmax, x0, xs);
        cff = cd_refpoly_ff(c, P_p_k, P_p_T, P_p_Tt, P_kr, P_Ti);
    end
    
    % Calculate the control signal and reference polynomial value based on current time
    if t >= te
        enable = false;
        w_p = polyval(c, te);
        u_vp1_t = polyval(cff, te);
    else
        enable = true;
        w_p = polyval(c, t);
        u_vp1_t = polyval(cff, t);
    end
end

== matlab function s9_template/control_software/v_max_switch ==
  data: pos_vmax input; v_ref output; vmax input; type input
function v_ref = v_max_switch(pos_vmax, vmax, type)
    % FCN - Calculates the reference velocity value based on the specified type.
    %
    % This function returns a reference velocity value depending on the type specified.
    % There are two possible reference velocities: a position-dependent maximum 
    % velocity (pos_vmax) and a fixed maximum velocity (vmax).
    %
    % Input parameters:
    % pos_vmax [m/s] - The position-dependent maximum velocity
    % vmax [m/s]   - The fixed maximum velocity
    % type [1]  - The type indicator, which determines which velocity is used as the reference
    %
    % Output parameter:
    % v_ref [m/s]  - The calculated reference velocity
    %
    % The function selects the reference velocity based on the value of 'type'.
    % If 'type' equals 1, 'pos_vmax' is used as the reference velocity;
    % otherwise, 'vmax' is used.
    if type == 1
        v_ref = pos_vmax;
    else
        v_ref = vmax;
    end
end

== matlab function s9_template/control_software/safety_halt ==
  data: carid input; cmd_old input; cmd output; pedals output; caroutputsext input; CarInputsCmdHalt parameter; a1total parameter; a2total parameter; P_safety_buffer parameter; P_prevent_buffer parameter; pedals_old input; steering_old input; steering output; activate input
function [cmd, pedals, steering] = safety_halt(carid, cmd_old, caroutputsext, CarInputsCmdHalt, a1total, a2total, P_safety_buffer, P_prevent_buffer, pedals_old, steering_old, activate)
    % SAFETY_HALT - Executes a safety halt based on provided inputs and safety conditions.
    %
    % This function is designed to ensure vehicle safety by dynamically adjusting 
    % the vehicle's command, pedal, and steering positions based on various 
    % parameters and safety buffers. It utilizes a combination of current vehicle 
    % states and predefined safety thresholds to make decisions.
    %
    % Input parameters:
    % carid           - The ID of the vehicle.
    % cmd_old         - The previous command issued to the vehicle.
    % caroutputsext   - Extended output data of the vehicle, containing state information.
    % CarInputsCmdHalt - Command to halt the vehicle.
    % a1total, a2total [m] - Total positional values used for calculation.
    % P_safety_buffer [m] - Safety buffer for positional calculations.
    % P_prevent_buffer [m] - Buffer for preventive measures.
    % pedals_old      - The previous state of the pedals.
    % steering_old    - The previous steering position.
    % activate        - Controls whether the function is active or not.
    %
    % Output parameters:
    % cmd             - The current command for the vehicle.
    % pedals          - The current state of the pedals.
    % steering        - The current steering position.
    %
    % The function operates with a persistent 'halt' state, which retains its value
    % across function calls. This state assists in determining whether to continue
    % halting the vehicle or return to previous commands and control states.
    %
    % The decision logic within the function includes checks for data validity,
    % adherence to positional thresholds, and adjustments based on the defined
    % safety and preventive buffers. These checks ensure the vehicle operates
    % within safe parameters, particularly in response to dynamic conditions.



    persistent halt; % Persistent variable to save the hold state between calls

    % Initialize 'halt' on first call
    if isempty(halt)
        halt = false;
    end

    if activate == 1
        % Check for data validity and basic conditions
        % Checks whether messages are lost and stops the car if this happens.
        if isempty(caroutputsext.s1) || isempty(caroutputsext.s2) || ...
           isempty(caroutputsext.psi) || isempty(caroutputsext.beta) || ...
           isempty(caroutputsext.x) || isempty(caroutputsext.v) || ...
           isempty(caroutputsext.time)
            cmd = CarInputsCmdHalt;
            halt = true;
        else
            % As soon as the car leaves the road, the car is permanently
            % stopped and transferred to a safe state
            if halt
                cmd = CarInputsCmdHalt;
            else
                cmd = cmd_old;
            end
        end

        % Additional checks based on positional thresholds
        % Checks whether the correct CARID is present or whether the car is 
        % outside the safety area; if this is the case, the car is stopped.
        if (carid ~= 0) || caroutputsext.s1 > (a1total - P_safety_buffer) || ...
           caroutputsext.s2 > (a2total - P_safety_buffer) || ...
           caroutputsext.s1 < (0 + P_safety_buffer) || ...
           caroutputsext.s2 < (0 + P_safety_buffer)
            pedals = 0.0;
            cmd = CarInputsCmdHalt;
            halt = true;
        end

        % Checks if the car is closer than 5 cm to the end of the road, if 
        % so the car is slowed down and an offset is added to the steering 
        % to get away from the end of the road as quickly as possible.
        if caroutputsext.s1 > (a1total - P_prevent_buffer) || ...
           caroutputsext.s2 > (a2total - P_prevent_buffer) || ...
           caroutputsext.s1 < (0 + P_prevent_buffer) || ...
           caroutputsext.s2 < (0 + P_prevent_buffer)
            pedals = 0.05;

            % Checks the steering and then adds an offset depending on the steering.
            if steering_old >= 0
                steering = steering_old + 0.10;
            else
                steering = steering_old - 0.10;
            end
        else

            steering = steering_old;
            pedals = pedals_old;
        end
    else
        % If the safty halt is not activated, the old sizes are passed on
        steering = steering_old;
        pedals = pedals_old;

        % As soon as the car leaves the road, the car is permanently
        % stopped and transferred to a safe state
        if halt
            cmd = CarInputsCmdHalt;
        else
            cmd = cmd_old;
        end
    end
end

== matlab function s9_template/control_software/pedals_constrain ==
  data: cmd input; pedals input; pedals output
function pedals = pedals_constrain(cmd, pedals)
    % FCN - Adjusts the pedal value based on the command and the current pedal value.
    %
    % This function receives a command value (cmd) and a current pedal value
    % (pedals), and adjusts the pedal value accordingly. The adjusted pedal
    % value is dependent on the command value and the limits of the pedal value.
    %
    % Input parameters:
    % cmd [1]    - The command value that controls the adjustment of the pedal value
    % pedals [1] - The current pedal value to be adjusted
    %
    % Output parameter:
    % pedals [1] - The adjusted pedal value
    %
    % The function modifies the pedal value within a specific range. If 'cmd' equals 2,
    % the pedal value is constrained between -1 and 0. For other 'cmd' values, 
    % the pedal value is constrained between 0 and 1.

    if cmd == 2
        if pedals < -1
            pedals = -1;
        elseif pedals>=0
            pedals = 0;
        else
            pedals = pedals;
        end
    else
        if pedals > 1
            pedals = 1;
        elseif pedals<=0
            pedals = 0;
        else
            pedals = pedals;
        end
    end
end

== matlab function s9_template/vehicle_dynamics/decision_logic_u_n ==
  data: u_cmd input; u_n input; u_n output; CarInputsCmdHalt parameter; CarInputsCmdForward parameter; CarInputsCmdReverse parameter
function u_n = decision_logic_u_n(u_cmd, u_n, CarInputsCmdHalt, CarInputsCmdForward, CarInputsCmdReverse)
    % Function: fcn
    % Description: Adjusts the motor control signal based on the current command and
    %              the car's current motor signal state.
    %
    % Inputs:
    %   u_cmd [1] - Current command to the car, dictating its intended movement or action.
    %   u_n [1] - Current motor control signal of the car.
    %   CarInputsCmdHalt [1] - Command value representing the 'Halt' action.
    %   CarInputsCmdForward [1] - Command value representing the 'Move Forward' action.
    %   CarInputsCmdReverse [1] - Command value representing the 'Move Reverse' action.
    %
    % Output:
    %   u_n [1] - Updated motor control signal after applying the command logic.
    %
    % The function updates the motor control signal based on the received command. If the command
    % is to halt, it sets the motor signal to zero. For forward or reverse commands, it adjusts
    % the motor signal appropriately, ensuring no reverse action if moving forward, and vice versa.
    % It also limits the motor signal to a maximum and minimum range.
   
    % Logic to determine the new motor control signal based on the command
    if (u_cmd == CarInputsCmdHalt)
        u_n = 0;
    elseif (u_cmd == CarInputsCmdForward && u_n < 0)
        u_n = 0;
    elseif (u_cmd == CarInputsCmdReverse && u_n > 0)
        u_n = 0;
    elseif u_cmd == CarInputsCmdForward && u_n > 1
        u_n = 1;
    elseif u_cmd == CarInputsCmdReverse && u_n < -1
        u_n = -1;
    else
        u_n = u_n;
    end
end

== matlab function s9_template/vehicle_dynamics/conv_to_cartesian ==
  data: s1_input input; y1 output; s2_input input; psi input; y2 output; P_p_lr parameter
function [y1, y2] = conv_to_cartesian(s1_input, s2_input, psi, P_p_lr)
    % Function: fcn
    % Description: Computes Cartesian coordinates by adjusting input coordinates
    %              with trigonometric transformations.
    %
    % Inputs:
    %   s1_input [1] - Initial x-coordinate or a similar parameter.
    %   s2_input [1] - Initial y-coordinate or a similar parameter.
    %   psi [rad]    - Angle in radians, used in the trigonometric transformations.
    %   P_p_lr [m]   - A distance or offset parameter influencing the calculation.
    %
    % Outputs:
    %   y1 [1] - The computed x-coordinate after applying the cosine transformation.
    %   y2 [1] - The computed y-coordinate after applying the sine transformation.
    %
    % The function calculates new Cartesian coordinates (y1, y2) by subtracting
    % the product of P_p_lr and the cosine (for y1) or sine (for y2) of the angle psi
    % from the input coordinates (s1_input, s2_input).
    
    % Calculation of the Cartesian coordinates
    y1 = s1_input - (P_p_lr * cos(psi));
    y2 = s2_input - (P_p_lr * sin(psi));
end

== matlab function s9_template/vehicle_dynamics/vehicle_dynamics_highspeed/calculate_alpha_r ==
  data: v_c1 input; alpha_r output; v_c2 input; psi_p input; P_p_lr parameter
function alpha_r = calculate_alpha_r(v_c1, v_c2, psi_p, P_p_lr)
    % Function: calculate_alpha_r
    % Description: Calculates the rear slip angle 'alpha_r' based on vehicle velocities
    %              and dynamics.
    %
    % Inputs:
    %   v_c1 [m/s] - Longitudinal component of the center of gravity (COG) velocity.
    %   v_c2 [m/s] - Lateral component of the COG velocity.
    %   psi_p [rad] - Yaw rate of the vehicle.
    %   P_p_lr [rad] - Distance from the COG to the rear axle.
    %
    % Output:
    %   alpha_r [rad] - Calculated rear slip angle considering the vehicle's dynamics.
    %
    % The function computes the rear slip angle 'alpha_r', taking into account the longitudinal 
    % and lateral velocities of the vehicle's COG, its yaw rate, and the distance from the COG 
    % to the rear axle. The calculation adjusts based on whether the longitudinal velocity 
    % component (v_c1) is positive, negative, or zero.
    
    % Calculation of the rear slip angle 'alpha_r'
    if (v_c1 > 0)
        alpha_r = -atan((v_c2 - (P_p_lr * psi_p)) / v_c1);
    elseif (v_c1 < 0)
        alpha_r = atan((v_c2 - (P_p_lr * psi_p)) / v_c1);
    else 
        alpha_r = 0;
    end
end

== matlab function s9_template/vehicle_dynamics/vehicle_dynamics_highspeed/calculate_alpha_f ==
  data: v_c1 input; alpha_f output; v_c2 input; psi_p input; delta input; P_p_lf parameter
function alpha_f = calculate_alpha_f(v_c1, v_c2, psi_p, delta, P_p_lf)
    % Function: calculate_alpha_f
    % Description: Calculates the angle 'alpha_f' based on vehicle dynamics and geometry.
    %
    % Inputs:
    %   v_c1 [m/s] - Longitudinal component of the center of gravity (COG) velocity.
    %   v_c2 [m/s] - Lateral component of the center of gravity (COG) velocity.
    %   psi_p [rad] - Yaw rate of the vehicle.
    %   delta [rad] - Steering angle.
    %   P_p_lf [m]-  Distance from the COG to the front axle.
    %
    % Output:
    %   alpha_f [rad] - Calculated angle factoring in vehicle dynamics and geometry.
    %
    % The function computes the angle 'alpha_f' considering the longitudinal and lateral 
    % components of the COG velocity, the vehicle's yaw rate, and steering angle. It takes 
    % into account the distance from the COG to the rear axle. The computation adjusts 
    % based on whether the longitudinal velocity component (v_c1) is positive, negative, 
    % or zero.

    % Calculation of the angle 'alpha_f'
    if (v_c1 > 0)
        alpha_f = -atan((v_c2 + (P_p_lf * psi_p)) / v_c1) + delta;
    elseif (v_c1 < 0)
        alpha_f = atan((v_c2 + (P_p_lf * psi_p)) / v_c1) - delta;
    else
        alpha_f = 0;
    end
end

== matlab function s9_template/vehicle_dynamics/vehicle_dynamics_highspeed/calculate_F_f_and_F_r ==
  data: F_f output; alpha_f input; alpha_r input; F_r output; P_p_Bf parameter; P_p_Cf parameter; P_p_Df parameter; P_p_Ef parameter; P_p_Br parameter; P_p_Cr parameter; P_p_Dr parameter; P_p_Er parameter
function [F_f, F_r] = calculate_F_f_and_F_r(alpha_f, alpha_r, P_p_Bf, P_p_Cf, P_p_Df, P_p_Ef, P_p_Br, P_p_Cr, P_p_Dr, P_p_Er)
    % Function: calculate_F_f_and_F_r
    % Description: Calculates the tire forces at the front (F_f) and rear (F_r) of the vehicle
    %              using the Magic Formula tire model.
    %
    % Inputs:
    %   alpha_f [rad] - Front slip angle.
    %   alpha_r [rad] - Rear slip angle.
    %   P_p_Bf, P_p_Cf, P_p_Df, P_p_Ef - Magic Formula coefficients for the front tire.
    %   P_p_Br, P_p_Cr, P_p_Dr, P_p_Er - Magic Formula coefficients for the rear tire.
    %
    % Outputs:
    %   F_f [N] - Calculated tire force at the front.
    %   F_r [N] - Calculated tire force at the rear.
    %
    % The function employs the Magic Formula to compute the tire forces at the front and rear
    % of the vehicle. These forces are crucial for analyzing vehicle dynamics, especially in
    % terms of handling and stability.

    % Calculation of the front and rear tire forces
    F_f = P_p_Df * sin(P_p_Cf * atan(P_p_Bf * (1 - P_p_Ef) * alpha_f - (P_p_Ef * atan(P_p_Bf * alpha_f))));
    F_r = P_p_Dr * sin(P_p_Cr * atan(P_p_Br * (1 - P_p_Er) * alpha_r - (P_p_Er * atan(P_p_Br * alpha_r))));
end
